simulink model "controller"  (R2018b)
settings: Solver=ode4  StartTime=0.0  StopTime=10.0  FixedStep=0.01  RelTol=1e-3
values from neighbouring files (symbols this model uses):
  K = 1000    [dane.m]
  T = 0.01    [dane.m]
  vmin = 1.4    [dane.m]
settings Model: Creator=lpa1  LastModifiedBy=User

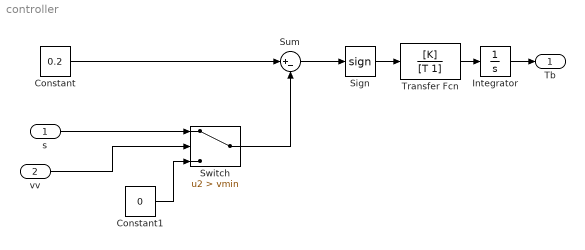
== system controller ==
  s : Inport
  "vv " : Inport  Port=2
  Constant : Constant  Value=0.2
  Constant1 : Constant  Value=0
  Integrator : Integrator
  Sign : Signum
  Sum : Sum  Inputs=|+-
  Switch : Switch  Criteria=u2 > Threshold  Threshold=vmin
  Transfer Fcn : TransferFcn  Numerator=[K]  Denominator=[T 1]
  Tb : Outport
  wires:
  Constant/1 -> Sum/1
  s/1 -> Switch/1
  Constant1/1 -> Switch/3
  "vv "/1 -> Switch/2
  Switch/1 -> Sum/2
  Sum/1 -> Sign/1
  Sign/1 -> Transfer Fcn/1
  Transfer Fcn/1 -> Integrator/1
  Integrator/1 -> Tb/1
